simulink model "tutorial39_top"  (R2025a)
settings: Solver=VariableStepAuto  StartTime=0.0  StopTime=10.0  RelTol=1e-3
settings Model: Creator=xing2  LastModifiedBy=xing2

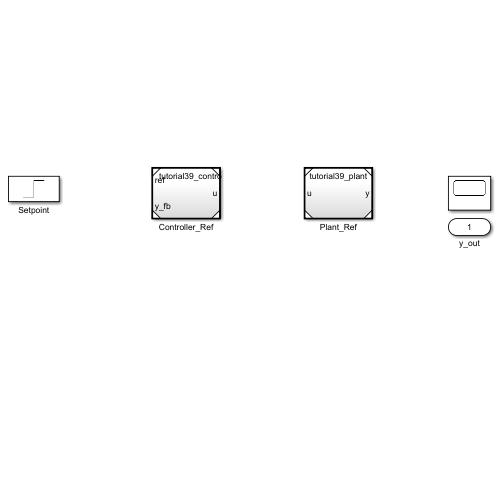
[thumbnail: Simulink's stored preview of the top-level diagram]
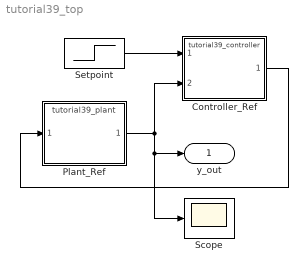
== system tutorial39_top ==
  Controller_Ref : ModelReference  ModelNameDialog=tutorial39_controller  SimulationMode=Normal  ModelReferenceVersion=1.1
  Plant_Ref : ModelReference  ModelNameDialog=tutorial39_plant  SimulationMode=Normal  ModelReferenceVersion=1.1
  Scope : Scope
  Setpoint : Step  Time=0.5  SampleTime=0
  y_out : Outport
  wires:
  Setpoint/1 -> Controller_Ref/1
  Controller_Ref/1 -> Plant_Ref/1
  Plant_Ref/1 -> Scope/1, y_out/1, Controller_Ref/2
